simulink model "MdEnChk6s7s_Caller"  (R2018b)
settings: Solver=FixedStepDiscrete  StartTime=0.0  StopTime=10.0  RelTol=1e-3
undefined symbols (not defined in the file or in its folder): ChkBsyBit, MdAvl, MdEnChk6s7s_MdXX_Cal, Req, SetBsyBit, SetEnBit
libraries: simulink x6
settings Model: Creator=sn2xws  LastModifiedBy=sn2xws
settings DataIOCC: SaveFormat=StructureWithTime
settings OptimizationCC: DefaultParameterBehavior=Inlined  EnhancedBackFolding=on  PassReuseOutputArgsAs=Individual arguments  ZeroExternalMemoryAtStartup=off  ZeroInternalMemoryAtStartup=off  OptimizeBlockOrder=speed  DifferentSizesBufferReuse=on  OptimizationCustomize=off
settings DebuggingCC: ParameterTunabilityLossMsg=error
settings SFSimCC: MATLABDynamicMemAlloc=off
settings RTWCC: SystemTargetFile=autosar.tlc  GenCodeOnly=on  TemplateMakefile=ert_default_tmf  Description=AUTOSAR  GenerateReport=on  IncludeHyperlinkInReport=on  LaunchReport=on  GenerateTraceInfo=on  GenerateTraceReport=on  GenerateTraceReportSl=on  GenerateTraceReportSf=on  GenerateTraceReportEml=on  GenerateCodeMetricsReport=on
settings CodeAppCC: ForceParamTrailComments=on  IgnoreCustomStorageClasses=off  OperatorAnnotations=on  SimulinkDataObjDesc=on  SFDataObjDesc=on  InsertBlockDesc=on
settings STFCustomTargetCC: TargetLangStandard=C99 (ISO)  MultiwordLength=256  ParMdlRefBuildCompliant=on  CompOptLevelCompliant=on  IncludeMdlTerminateFcn=off  CombineOutputUpdateFcns=on  SuppressErrorStatus=on  ERTCustomFileBanners=on  SupportNonFinite=off  SupportComplex=off  SupportContinuousTime=off  SupportNonInlinedSFcns=off  RemoveResetFunc=on  MATLABClassNameForMDSCustomization=Simulink.SoftwareTarget.ERTCustomization  AutosarCompliant=on  UseToolchainInfoCompliant=on  LookupTableObjectStructAxisOrder=2,1,3,4,...  LUTObjectStructOrderEvenSpacing=Size,Table,Breakpoints  SystemTargetFile=autosar.tlc
settings ERTTargetCC: TargetLangStandard=C99 (ISO)  ConcurrentExecutionCompliant=off  IncludeMdlTerminateFcn=off  SuppressErrorStatus=on  SupportNonFinite=off  SupportComplex=off  ModelStepFunctionPrototypeControlCompliant=off  CPPClassGenCompliant=off  AutosarCompliant=on  LookupTableObjectStructAxisOrder=2,1,3,4,...  LUTObjectStructOrderEvenSpacing=Size,Table,Breakpoints  InlinedParameterPlacement=NonHierarchical  ERTCustomFileTemplate=example_file_process.tlc  ERTFilePackagingFormat=Compact

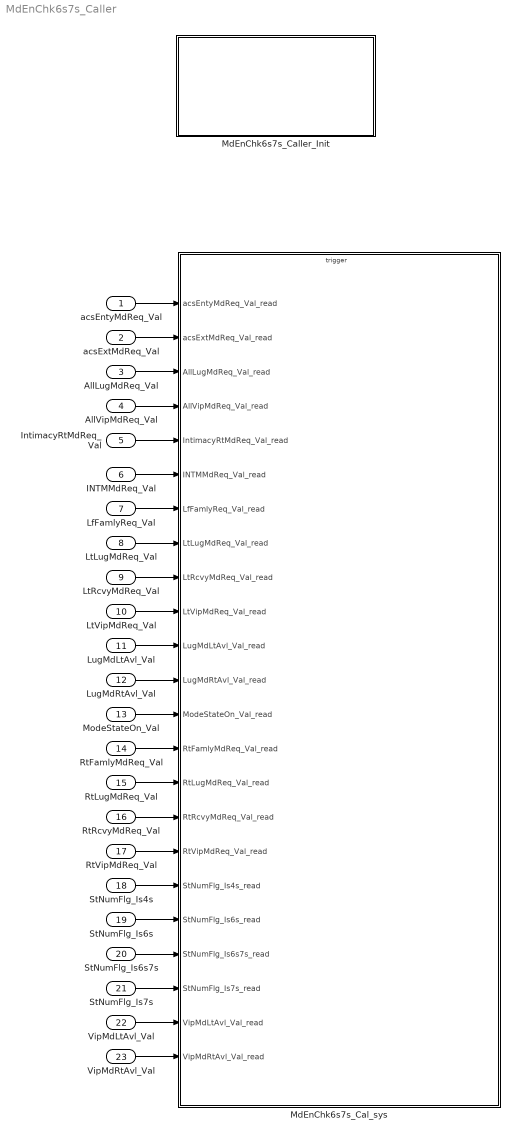
== system MdEnChk6s7s_Caller ==
  acsEntyMdReq_Val : Inport  OutDataTypeStr=boolean  PortDimensions=1
  acsExtMdReq_Val : Inport  Port=2  OutDataTypeStr=boolean  PortDimensions=1
  AllLugMdReq_Val : Inport  Port=3  OutDataTypeStr=boolean  PortDimensions=1
  AllVipMdReq_Val : Inport  Port=4  OutDataTypeStr=boolean  PortDimensions=1
  IntimacyRtMdReq_Val : Inport  Port=5  OutDataTypeStr=boolean  PortDimensions=1
  INTMMdReq_Val : Inport  Port=6  OutDataTypeStr=boolean  PortDimensions=1
  LfFamlyReq_Val : Inport  Port=7  OutDataTypeStr=boolean  PortDimensions=1
  LtLugMdReq_Val : Inport  Port=8  OutDataTypeStr=boolean  PortDimensions=1
  LtRcvyMdReq_Val : Inport  Port=9  OutDataTypeStr=boolean  PortDimensions=1
  LtVipMdReq_Val : Inport  Port=10  OutDataTypeStr=boolean  PortDimensions=1
  LugMdLtAvl_Val : Inport  Port=11  OutDataTypeStr=boolean  PortDimensions=1
  LugMdRtAvl_Val : Inport  Port=12  OutDataTypeStr=boolean  PortDimensions=1
  ModeStateOn_Val : Inport  Port=13  OutDataTypeStr=boolean  PortDimensions=1
  RtFamlyMdReq_Val : Inport  Port=14  OutDataTypeStr=boolean  PortDimensions=1
  RtLugMdReq_Val : Inport  Port=15  OutDataTypeStr=boolean  PortDimensions=1
  RtRcvyMdReq_Val : Inport  Port=16  OutDataTypeStr=boolean  PortDimensions=1
  RtVipMdReq_Val : Inport  Port=17  OutDataTypeStr=boolean  PortDimensions=1
  StNumFlg_Is4s : Inport  Port=18  OutDataTypeStr=boolean  PortDimensions=1
  StNumFlg_Is6s : Inport  Port=19  OutDataTypeStr=boolean  PortDimensions=1
  StNumFlg_Is6s7s : Inport  Port=20  OutDataTypeStr=boolean  PortDimensions=1
  StNumFlg_Is7s : Inport  Port=21  OutDataTypeStr=boolean  PortDimensions=1
  VipMdLtAvl_Val : Inport  Port=22  OutDataTypeStr=boolean  PortDimensions=1
  VipMdRtAvl_Val : Inport  Port=23  OutDataTypeStr=boolean  PortDimensions=1
  MdEnChk6s7s_Cal_sys : Subsystem
  MdEnChk6s7s_Caller_Init : Subsystem
  wires:
  acsEntyMdReq_Val/1 -> MdEnChk6s7s_Cal_sys/1(acsEntyMdReq_Val_read)
  acsExtMdReq_Val/1 -> MdEnChk6s7s_Cal_sys/2(acsExtMdReq_Val_read)
  AllLugMdReq_Val/1 -> MdEnChk6s7s_Cal_sys/3(AllLugMdReq_Val_read)
  AllVipMdReq_Val/1 -> MdEnChk6s7s_Cal_sys/4(AllVipMdReq_Val_read)
  IntimacyRtMdReq_Val/1 -> MdEnChk6s7s_Cal_sys/5(IntimacyRtMdReq_Val_read)
  INTMMdReq_Val/1 -> MdEnChk6s7s_Cal_sys/6(INTMMdReq_Val_read)
  LfFamlyReq_Val/1 -> MdEnChk6s7s_Cal_sys/7(LfFamlyReq_Val_read)
  LtLugMdReq_Val/1 -> MdEnChk6s7s_Cal_sys/8(LtLugMdReq_Val_read)
  LtRcvyMdReq_Val/1 -> MdEnChk6s7s_Cal_sys/9(LtRcvyMdReq_Val_read)
  LtVipMdReq_Val/1 -> MdEnChk6s7s_Cal_sys/10(LtVipMdReq_Val_read)
  LugMdLtAvl_Val/1 -> MdEnChk6s7s_Cal_sys/11(LugMdLtAvl_Val_read)
  LugMdRtAvl_Val/1 -> MdEnChk6s7s_Cal_sys/12(LugMdRtAvl_Val_read)
  ModeStateOn_Val/1 -> MdEnChk6s7s_Cal_sys/13(ModeStateOn_Val_read)
  RtFamlyMdReq_Val/1 -> MdEnChk6s7s_Cal_sys/14(RtFamlyMdReq_Val_read)
  RtLugMdReq_Val/1 -> MdEnChk6s7s_Cal_sys/15(RtLugMdReq_Val_read)
  RtRcvyMdReq_Val/1 -> MdEnChk6s7s_Cal_sys/16(RtRcvyMdReq_Val_read)
  RtVipMdReq_Val/1 -> MdEnChk6s7s_Cal_sys/17(RtVipMdReq_Val_read)
  StNumFlg_Is4s/1 -> MdEnChk6s7s_Cal_sys/18(StNumFlg_Is4s_read)
  StNumFlg_Is6s/1 -> MdEnChk6s7s_Cal_sys/19(StNumFlg_Is6s_read)
  StNumFlg_Is6s7s/1 -> MdEnChk6s7s_Cal_sys/20(StNumFlg_Is6s7s_read)
  StNumFlg_Is7s/1 -> MdEnChk6s7s_Cal_sys/21(StNumFlg_Is7s_read)
  VipMdLtAvl_Val/1 -> MdEnChk6s7s_Cal_sys/22(VipMdLtAvl_Val_read)
  VipMdRtAvl_Val/1 -> MdEnChk6s7s_Cal_sys/23(VipMdRtAvl_Val_read)

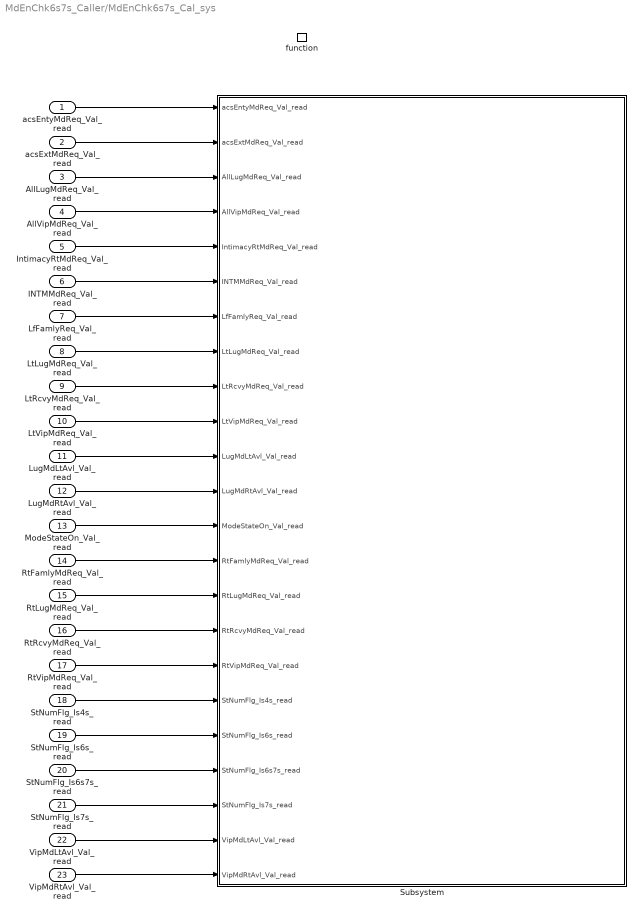
== system MdEnChk6s7s_Caller/MdEnChk6s7s_Cal_sys ==
  acsEntyMdReq_Val_read : Inport
  acsExtMdReq_Val_read : Inport  Port=2
  AllLugMdReq_Val_read : Inport  Port=3
  AllVipMdReq_Val_read : Inport  Port=4
  IntimacyRtMdReq_Val_read : Inport  Port=5
  INTMMdReq_Val_read : Inport  Port=6
  LfFamlyReq_Val_read : Inport  Port=7
  LtLugMdReq_Val_read : Inport  Port=8
  LtRcvyMdReq_Val_read : Inport  Port=9
  LtVipMdReq_Val_read : Inport  Port=10
  LugMdLtAvl_Val_read : Inport  Port=11
  LugMdRtAvl_Val_read : Inport  Port=12
  ModeStateOn_Val_read : Inport  Port=13
  RtFamlyMdReq_Val_read : Inport  Port=14
  RtLugMdReq_Val_read : Inport  Port=15
  RtRcvyMdReq_Val_read : Inport  Port=16
  RtVipMdReq_Val_read : Inport  Port=17
  StNumFlg_Is4s_read : Inport  Port=18
  StNumFlg_Is6s_read : Inport  Port=19
  StNumFlg_Is6s7s_read : Inport  Port=20
  StNumFlg_Is7s_read : Inport  Port=21
  VipMdLtAvl_Val_read : Inport  Port=22
  VipMdRtAvl_Val_read : Inport  Port=23
  function : TriggerPort  TriggerType=function-call  IsSimulinkFunction=on  FunctionName=MdEnChk6s7s_Cal  VariantControl=(inherit)
  Subsystem : Subsystem
  wires:
  acsEntyMdReq_Val_read/1 -> Subsystem/1(acsEntyMdReq_Val_read)
  acsExtMdReq_Val_read/1 -> Subsystem/2(acsExtMdReq_Val_read)
  AllLugMdReq_Val_read/1 -> Subsystem/3(AllLugMdReq_Val_read)
  AllVipMdReq_Val_read/1 -> Subsystem/4(AllVipMdReq_Val_read)
  IntimacyRtMdReq_Val_read/1 -> Subsystem/5(IntimacyRtMdReq_Val_read)
  INTMMdReq_Val_read/1 -> Subsystem/6(INTMMdReq_Val_read)
  LfFamlyReq_Val_read/1 -> Subsystem/7(LfFamlyReq_Val_read)
  LtLugMdReq_Val_read/1 -> Subsystem/8(LtLugMdReq_Val_read)
  LtRcvyMdReq_Val_read/1 -> Subsystem/9(LtRcvyMdReq_Val_read)
  LtVipMdReq_Val_read/1 -> Subsystem/10(LtVipMdReq_Val_read)
  LugMdLtAvl_Val_read/1 -> Subsystem/11(LugMdLtAvl_Val_read)
  LugMdRtAvl_Val_read/1 -> Subsystem/12(LugMdRtAvl_Val_read)
  ModeStateOn_Val_read/1 -> Subsystem/13(ModeStateOn_Val_read)
  RtFamlyMdReq_Val_read/1 -> Subsystem/14(RtFamlyMdReq_Val_read)
  RtLugMdReq_Val_read/1 -> Subsystem/15(RtLugMdReq_Val_read)
  RtRcvyMdReq_Val_read/1 -> Subsystem/16(RtRcvyMdReq_Val_read)
  RtVipMdReq_Val_read/1 -> Subsystem/17(RtVipMdReq_Val_read)
  StNumFlg_Is4s_read/1 -> Subsystem/18(StNumFlg_Is4s_read)
  StNumFlg_Is6s_read/1 -> Subsystem/19(StNumFlg_Is6s_read)
  StNumFlg_Is6s7s_read/1 -> Subsystem/20(StNumFlg_Is6s7s_read)
  StNumFlg_Is7s_read/1 -> Subsystem/21(StNumFlg_Is7s_read)
  VipMdLtAvl_Val_read/1 -> Subsystem/22(VipMdLtAvl_Val_read)
  VipMdRtAvl_Val_read/1 -> Subsystem/23(VipMdRtAvl_Val_read)

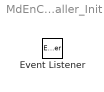
== system MdEnChk6s7s_Caller/MdEnChk6s7s_Caller_Init ==
  Event Listener : EventListener  EventName=reset

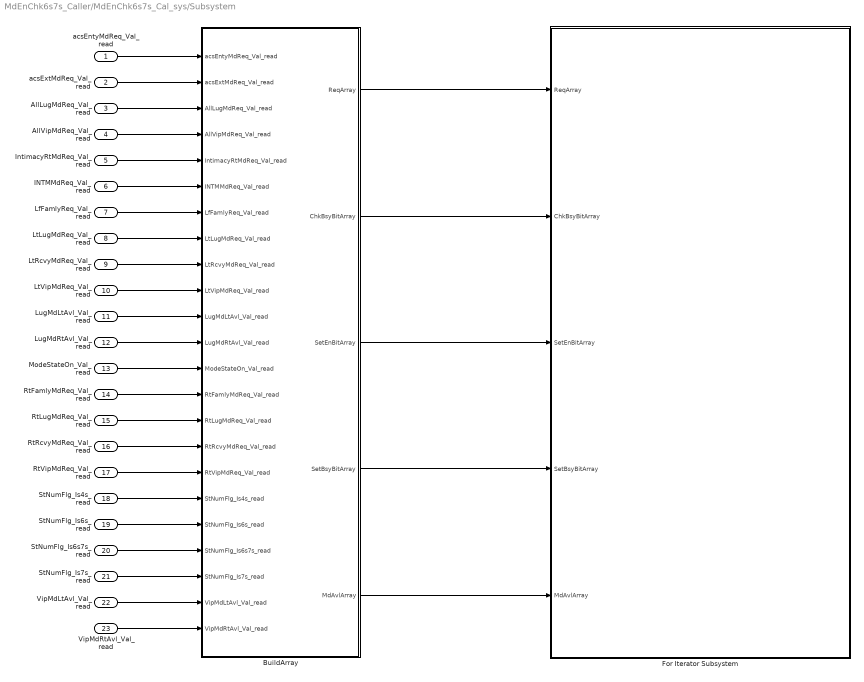
== system MdEnChk6s7s_Caller/MdEnChk6s7s_Cal_sys/Subsystem ==
  acsEntyMdReq_Val_read : Inport
  acsExtMdReq_Val_read : Inport  Port=2
  AllLugMdReq_Val_read : Inport  Port=3
  AllVipMdReq_Val_read : Inport  Port=4
  IntimacyRtMdReq_Val_read : Inport  Port=5
  INTMMdReq_Val_read : Inport  Port=6
  LfFamlyReq_Val_read : Inport  Port=7
  LtLugMdReq_Val_read : Inport  Port=8
  LtRcvyMdReq_Val_read : Inport  Port=9
  LtVipMdReq_Val_read : Inport  Port=10
  LugMdLtAvl_Val_read : Inport  Port=11
  LugMdRtAvl_Val_read : Inport  Port=12
  ModeStateOn_Val_read : Inport  Port=13
  RtFamlyMdReq_Val_read : Inport  Port=14
  RtLugMdReq_Val_read : Inport  Port=15
  RtRcvyMdReq_Val_read : Inport  Port=16
  RtVipMdReq_Val_read : Inport  Port=17
  StNumFlg_Is4s_read : Inport  Port=18
  StNumFlg_Is6s_read : Inport  Port=19
  StNumFlg_Is6s7s_read : Inport  Port=20
  StNumFlg_Is7s_read : Inport  Port=21
  VipMdLtAvl_Val_read : Inport  Port=22
  VipMdRtAvl_Val_read : Inport  Port=23
  BuildArray : Subsystem
  For Iterator Subsystem : Subsystem  TreatAsAtomicUnit=on
  wires:
  acsEntyMdReq_Val_read/1 -> BuildArray/1(acsEntyMdReq_Val_read)
  acsExtMdReq_Val_read/1 -> BuildArray/2(acsExtMdReq_Val_read)
  AllLugMdReq_Val_read/1 -> BuildArray/3(AllLugMdReq_Val_read)
  AllVipMdReq_Val_read/1 -> BuildArray/4(AllVipMdReq_Val_read)
  IntimacyRtMdReq_Val_read/1 -> BuildArray/5(IntimacyRtMdReq_Val_read)
  INTMMdReq_Val_read/1 -> BuildArray/6(INTMMdReq_Val_read)
  LfFamlyReq_Val_read/1 -> BuildArray/7(LfFamlyReq_Val_read)
  LtLugMdReq_Val_read/1 -> BuildArray/8(LtLugMdReq_Val_read)
  LtRcvyMdReq_Val_read/1 -> BuildArray/9(LtRcvyMdReq_Val_read)
  LtVipMdReq_Val_read/1 -> BuildArray/10(LtVipMdReq_Val_read)
  LugMdLtAvl_Val_read/1 -> BuildArray/11(LugMdLtAvl_Val_read)
  LugMdRtAvl_Val_read/1 -> BuildArray/12(LugMdRtAvl_Val_read)
  ModeStateOn_Val_read/1 -> BuildArray/13(ModeStateOn_Val_read)
  RtFamlyMdReq_Val_read/1 -> BuildArray/14(RtFamlyMdReq_Val_read)
  RtLugMdReq_Val_read/1 -> BuildArray/15(RtLugMdReq_Val_read)
  RtRcvyMdReq_Val_read/1 -> BuildArray/16(RtRcvyMdReq_Val_read)
  RtVipMdReq_Val_read/1 -> BuildArray/17(RtVipMdReq_Val_read)
  StNumFlg_Is4s_read/1 -> BuildArray/18(StNumFlg_Is4s_read)
  StNumFlg_Is6s_read/1 -> BuildArray/19(StNumFlg_Is6s_read)
  StNumFlg_Is6s7s_read/1 -> BuildArray/20(StNumFlg_Is6s7s_read)
  StNumFlg_Is7s_read/1 -> BuildArray/21(StNumFlg_Is7s_read)
  VipMdLtAvl_Val_read/1 -> BuildArray/22(VipMdLtAvl_Val_read)
  VipMdRtAvl_Val_read/1 -> BuildArray/23(VipMdRtAvl_Val_read)
  BuildArray/1(ReqArray) -> For Iterator Subsystem/1(ReqArray)
  BuildArray/2(ChkBsyBitArray) -> For Iterator Subsystem/2(ChkBsyBitArray)
  BuildArray/3(SetEnBitArray) -> For Iterator Subsystem/3(SetEnBitArray)
  BuildArray/4(SetBsyBitArray) -> For Iterator Subsystem/4(SetBsyBitArray)
  BuildArray/5(MdAvlArray) -> For Iterator Subsystem/5(MdAvlArray)

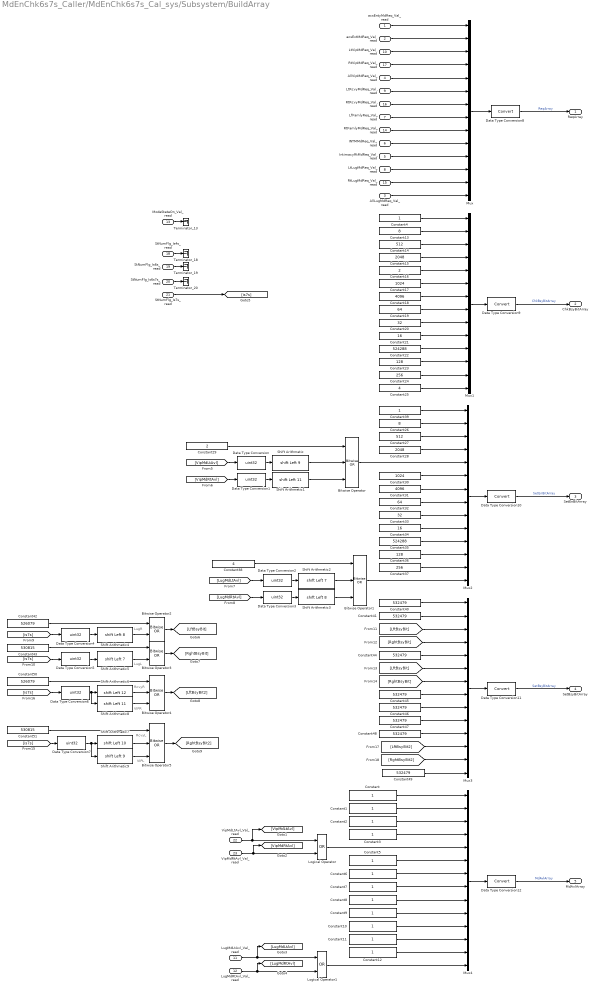
== system MdEnChk6s7s_Caller/MdEnChk6s7s_Cal_sys/Subsystem/BuildArray ==
  note: VIPR
  note: RcvyL
  note: VIPL
  note: RcvyR
  note: LugL
  note: LugR
  acsEntyMdReq_Val_read : Inport
  acsExtMdReq_Val_read : Inport  Port=2
  AllLugMdReq_Val_read : Inport  Port=3
  AllVipMdReq_Val_read : Inport  Port=4
  IntimacyRtMdReq_Val_read : Inport  Port=5
  INTMMdReq_Val_read : Inport  Port=6
  LfFamlyReq_Val_read : Inport  Port=7
  LtLugMdReq_Val_read : Inport  Port=8
  LtRcvyMdReq_Val_read : Inport  Port=9
  LtVipMdReq_Val_read : Inport  Port=10
  LugMdLtAvl_Val_read : Inport  Port=11
  LugMdRtAvl_Val_read : Inport  Port=12
  ModeStateOn_Val_read : Inport  Port=13
  RtFamlyMdReq_Val_read : Inport  Port=14
  RtLugMdReq_Val_read : Inport  Port=15
  RtRcvyMdReq_Val_read : Inport  Port=16
  RtVipMdReq_Val_read : Inport  Port=17
  StNumFlg_Is4s_read : Inport  Port=18
  StNumFlg_Is6s_read : Inport  Port=19
  StNumFlg_Is6s7s_read : Inport  Port=20
  StNumFlg_Is7s_read : Inport  Port=21
  VipMdLtAvl_Val_read : Inport  Port=22
  VipMdRtAvl_Val_read : Inport  Port=23
  Bitwise Operator{,1,4..5} (4 alike) : simulink/Logic and Bit Operations/Bitwise Operator  logicop=OR  UseBitMask=off  NumInputPorts=3  BitMask=bin2dec('11011001')  BitMaskRealWorld=Stored Integer
  Bitwise Operator2 : simulink/Logic and Bit Operations/Bitwise Operator  logicop=OR  UseBitMask=off  NumInputPorts=2  BitMask=bin2dec('11011001')  BitMaskRealWorld=Stored Integer
  Bitwise Operator3 : simulink/Logic and Bit Operations/Bitwise Operator  logicop=OR  UseBitMask=off  NumInputPorts=2  BitMask=bin2dec('11011001')  BitMaskRealWorld=Stored Integer
  Constant{,1..3,5..12} (12 alike) : Constant  OutDataTypeStr=boolean
  Constant13 : Constant  Value=8  OutDataTypeStr=uint32
  Constant14 : Constant  Value=512  OutDataTypeStr=uint32
  Constant15 : Constant  Value=2048  OutDataTypeStr=uint32
  Constant16 : Constant  Value=2  OutDataTypeStr=uint32
  Constant17 : Constant  Value=1024  OutDataTypeStr=uint32
  Constant18 : Constant  Value=4096  OutDataTypeStr=uint32
  Constant19 : Constant  Value=64  OutDataTypeStr=uint32
  Constant20 : Constant  Value=32  OutDataTypeStr=uint32
  Constant21 : Constant  Value=16  OutDataTypeStr=uint32
  Constant22 : Constant  Value=524288  OutDataTypeStr=uint32
  Constant23 : Constant  Value=128  OutDataTypeStr=uint32
  Constant24 : Constant  Value=256  OutDataTypeStr=uint32
  Constant25 : Constant  Value=4  OutDataTypeStr=uint32
  Constant26 : Constant  Value=8  OutDataTypeStr=uint32
  Constant27 : Constant  Value=512  OutDataTypeStr=uint32
  Constant28 : Constant  Value=2048  OutDataTypeStr=uint32
  Constant29 : Constant  Value=2  OutDataTypeStr=uint32
  Constant30 : Constant  Value=1024  OutDataTypeStr=uint32
  Constant31 : Constant  Value=4096  OutDataTypeStr=uint32
  Constant32 : Constant  Value=64  OutDataTypeStr=uint32
  Constant33 : Constant  Value=32  OutDataTypeStr=uint32
  Constant34 : Constant  Value=16  OutDataTypeStr=uint32
  Constant35 : Constant  Value=524288  OutDataTypeStr=uint32
  Constant36 : Constant  Value=128  OutDataTypeStr=uint32
  Constant37 : Constant  Value=256  OutDataTypeStr=uint32
  Constant38 : Constant  Value=4  OutDataTypeStr=uint32
  Constant39 : Constant  OutDataTypeStr=uint32
  Constant4 : Constant  OutDataTypeStr=uint32
  Constant{40..41,44..49} (8 alike) : Constant  Value=532479  OutDataTypeStr=uint32
  Constant42 : Constant  Value=526079  OutDataTypeStr=uint32
  Constant43 : Constant  Value=530815  OutDataTypeStr=uint32
  Constant50 : Constant  Value=526079  OutDataTypeStr=uint32
  Constant51 : Constant  Value=530815  OutDataTypeStr=uint32
  Data Type Conversion{,1..7} (8 alike) : DataTypeConversion  OutDataTypeStr=uint32
  Data Type Conversion{8..12} (5 alike) : DataTypeConversion
  Logical Operator : Logic  Operator=OR  AllPortsSameDT=off  OutDataTypeStr=boolean
  Logical Operator1 : Logic  Operator=OR  AllPortsSameDT=off  OutDataTypeStr=boolean
  Mux{,1..4} (5 alike) : Mux  Inputs=14
  Shift Arithmetic : ArithShift  BitShiftNumber=9  BitShiftDirection=Left
  Shift Arithmetic1 : ArithShift  BitShiftNumber=11  BitShiftDirection=Left
  Shift Arithmetic2 : ArithShift  BitShiftNumber=7  BitShiftDirection=Left
  Shift Arithmetic3 : ArithShift  BitShiftNumber=8  BitShiftDirection=Left
  Shift Arithmetic4 : ArithShift  BitShiftNumber=8  BitShiftDirection=Left
  Shift Arithmetic5 : ArithShift  BitShiftNumber=7  BitShiftDirection=Left
  Shift Arithmetic6 : ArithShift  BitShiftNumber=12  BitShiftDirection=Left
  Shift Arithmetic7 : ArithShift  BitShiftNumber=10  BitShiftDirection=Left
  Shift Arithmetic8 : ArithShift  BitShiftNumber=11  BitShiftDirection=Left
  Shift Arithmetic9 : ArithShift  BitShiftNumber=9  BitShiftDirection=Left
  Terminator_{13,18..20} (4 alike) : Terminator
  ReqArray : Outport
  ChkBsyBitArray : Outport  Port=2
  SetEnBitArray : Outport  Port=3
  SetBsyBitArray : Outport  Port=4
  MdAvlArray : Outport  Port=5
  wires:
  Constant43/1 -> Bitwise Operator3/1
  Shift Arithmetic5/1 -> Bitwise Operator3/2
  Constant42/1 -> Bitwise Operator2/1
  [LftBsyBit] -> Mux3/3
  Constant2/1 -> Mux4/3
  [RghtBsyBit2] -> Mux3/13
  Data Type Conversion3/1 -> Shift Arithmetic3/1
  Bitwise Operator2/1 -> [LftBsyBit]
  StNumFlg_Is7s_read/1 -> [is7s]
  Bitwise Operator5/1 -> [RghtBsyBit2]
  [LugMdRtAvl] -> Data Type Conversion3/1
  Constant12/1 -> Mux4/13
  [LugMdLtAvl] -> Data Type Conversion2/1
  Constant10/1 -> Mux4/11
  Constant8/1 -> Mux4/9
  Constant7/1 -> Mux4/8
  Constant6/1 -> Mux4/7
  Constant24/1 -> Mux1/13
  Constant25/1 -> Mux1/14
  Constant23/1 -> Mux1/12
  Constant22/1 -> Mux1/11
  Constant21/1 -> Mux1/10
  Constant20/1 -> Mux1/9
  Constant19/1 -> Mux1/8
  Constant18/1 -> Mux1/7
  Constant17/1 -> Mux1/6
  Constant15/1 -> Mux1/4
  Constant16/1 -> Mux1/5
  Constant14/1 -> Mux1/3
  [LftBsyBit2] -> Mux3/12
  IntimacyRtMdReq_Val_read/1 -> Mux/11
  acsExtMdReq_Val_read/1 -> Mux/2
  LfFamlyReq_Val_read/1 -> Mux/8
  Constant/1 -> Mux4/1
  Constant40/1 -> Mux3/1
  [RghtBsyBit] -> Mux3/4
  Shift Arithmetic6/1 -> Bitwise Operator4/2
  Mux3/1 -> Data Type Conversion11/1
  Constant49/1 -> Mux3/14
  Shift Arithmetic3/1 -> Bitwise Operator1/3
  Shift Arithmetic2/1 -> Bitwise Operator1/2
  Data Type Conversion5/1 -> Shift Arithmetic5/1
  VipMdLtAvl_Val_read/1 -> [VipMdLtAvl], Logical Operator/1
  Logical Operator/1 -> Mux4/5
  Logical Operator1/1 -> Mux4/14
  Bitwise Operator4/1 -> [LftBsyBit2]
  StNumFlg_Is6s_read/1 -> Terminator_19/1
  StNumFlg_Is4s_read/1 -> Terminator_18/1
  ModeStateOn_Val_read/1 -> Terminator_13/1
  Constant47/1 -> Mux3/10
  Constant1/1 -> Mux4/2
  StNumFlg_Is6s7s_read/1 -> Terminator_20/1
  Constant3/1 -> Mux4/4
  Data Type Conversion4/1 -> Shift Arithmetic4/1
  [LftBsyBit] -> Mux3/6
  RtRcvyMdReq_Val_read/1 -> Mux/7
  Mux2/1 -> Data Type Conversion10/1
  [RghtBsyBit] -> Mux3/7
  Constant38/1 -> Bitwise Operator1/1
  LtVipMdReq_Val_read/1 -> Mux/3
  RtVipMdReq_Val_read/1 -> Mux/4
  RtLugMdReq_Val_read/1 -> Mux/13
  LugMdLtAvl_Val_read/1 -> [LugMdLtAvl], Logical Operator1/1
  Constant29/1 -> Bitwise Operator/1
  Bitwise Operator/1 -> Mux2/5
  Shift Arithmetic1/1 -> Bitwise Operator/3
  Shift Arithmetic/1 -> Bitwise Operator/2
  [is7s] -> Data Type Conversion5/1
  AllLugMdReq_Val_read/1 -> Mux/14
  LtRcvyMdReq_Val_read/1 -> Mux/6
  Mux4/1 -> Data Type Conversion12/1
  LtLugMdReq_Val_read/1 -> Mux/12
  [is7s] -> Data Type Conversion6/1
  Bitwise Operator3/1 -> [RghtBsyBit]
  Bitwise Operator1/1 -> Mux2/14
  RtFamlyMdReq_Val_read/1 -> Mux/9
  Shift Arithmetic7/1 -> Bitwise Operator5/2
  Data Type Conversion7/1 -> Shift Arithmetic9/1, Shift Arithmetic7/1
  Shift Arithmetic9/1 -> Bitwise Operator5/3
  VipMdRtAvl_Val_read/1 -> Logical Operator/2, [VipMdRtAvl]
  Constant45/1 -> Mux3/8
  Constant9/1 -> Mux4/10
  Data Type Conversion2/1 -> Shift Arithmetic2/1
  Constant51/1 -> Bitwise Operator5/1
  Constant41/1 -> Mux3/2
  Constant11/1 -> Mux4/12
  acsEntyMdReq_Val_read/1 -> Mux/1
  [VipMdRtAvl] -> Data Type Conversion1/1
  Constant48/1 -> Mux3/11
  Constant46/1 -> Mux3/9
  Constant50/1 -> Bitwise Operator4/1
  Constant4/1 -> Mux1/1
  Shift Arithmetic8/1 -> Bitwise Operator4/3
  Data Type Conversion6/1 -> Shift Arithmetic8/1, Shift Arithmetic6/1
  Data Type Conversion/1 -> Shift Arithmetic/1
  AllVipMdReq_Val_read/1 -> Mux/5
  [is7s] -> Data Type Conversion4/1
  [VipMdLtAvl] -> Data Type Conversion/1
  Constant34/1 -> Mux2/10
  LugMdRtAvl_Val_read/1 -> [LugMdRtAvl], Logical Operator1/2
  Mux1/1 -> Data Type Conversion9/1
  Constant31/1 -> Mux2/7
  Constant35/1 -> Mux2/11
  Constant33/1 -> Mux2/9
  Constant27/1 -> Mux2/3
  Data Type Conversion1/1 -> Shift Arithmetic1/1
  Constant36/1 -> Mux2/12
  Constant32/1 -> Mux2/8
  Constant28/1 -> Mux2/4
  Constant37/1 -> Mux2/13
  Constant26/1 -> Mux2/2
  Constant5/1 -> Mux4/6
  Constant13/1 -> Mux1/2
  Constant39/1 -> Mux2/1
  INTMMdReq_Val_read/1 -> Mux/10
  Constant44/1 -> Mux3/5
  Constant30/1 -> Mux2/6
  Shift Arithmetic4/1 -> Bitwise Operator2/2
  [is7s] -> Data Type Conversion7/1
  Mux/1 -> Data Type Conversion8/1
  Data Type Conversion8/1 -> ReqArray/1  "ReqArray"
  Data Type Conversion9/1 -> ChkBsyBitArray/1  "ChkBsyBitArray"
  Data Type Conversion10/1 -> SetEnBitArray/1  "SetEnBitArray"
  Data Type Conversion11/1 -> SetBsyBitArray/1  "SetBsyBitArray"
  Data Type Conversion12/1 -> MdAvlArray/1  "MdAvlArray"

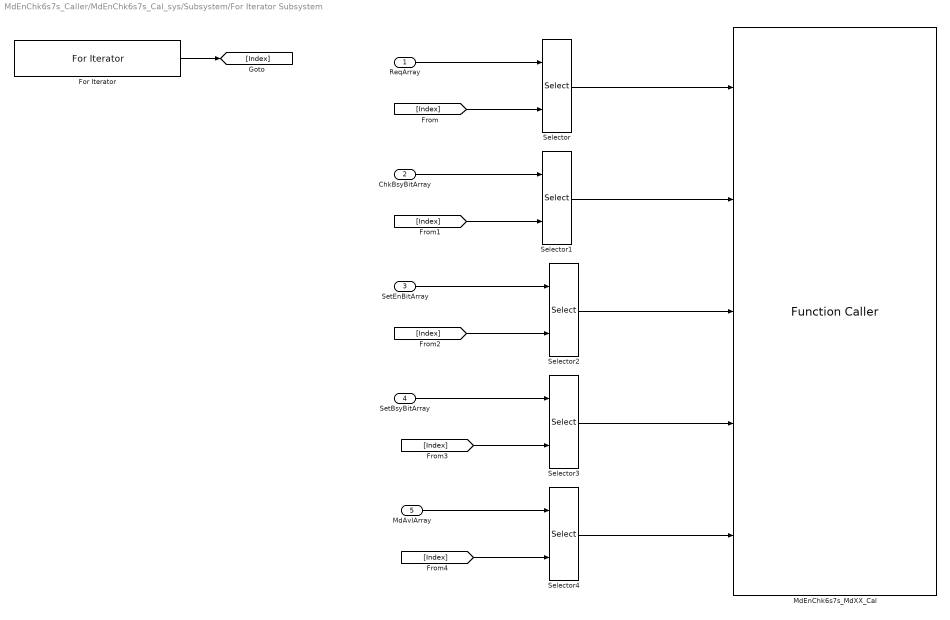
== system MdEnChk6s7s_Caller/MdEnChk6s7s_Cal_sys/Subsystem/For Iterator Subsystem ==
  ReqArray : Inport
  ChkBsyBitArray : Inport  Port=2
  SetEnBitArray : Inport  Port=3
  SetBsyBitArray : Inport  Port=4
  MdAvlArray : Inport  Port=5
  For Iterator : ForIterator  IterationLimit=14  IndexMode=Zero-based  IterationVariableDataType=int8
  MdEnChk6s7s_MdXX_Cal : FunctionCaller  Description=|  FunctionPrototype=MdEnChk6s7s_MdXX_Cal(Req,ChkBsyBit,SetEnBit,SetBsyBit,MdAvl)  InputArgumentSpecifications=boolean(true), uint32(1), uint32(1), uint32(1), boolean(true)
      | StNun: 
      | 0 :4s
      | 1:6s
      | 2:7s
      | 3:4sp
  Selector{,1..4} (5 alike) : Selector  IndexMode=Zero-based  InputPortWidth=14  IndexOptions=Index vector (port)  Indices=[1 3]  OutputSizes=1
  wires:
  For Iterator/1 -> [Index]
  [Index] -> Selector/2
  Selector/1 -> MdEnChk6s7s_MdXX_Cal/1
  [Index] -> Selector1/2
  Selector1/1 -> MdEnChk6s7s_MdXX_Cal/2
  Selector2/1 -> MdEnChk6s7s_MdXX_Cal/3
  [Index] -> Selector2/2
  [Index] -> Selector3/2
  [Index] -> Selector4/2
  Selector4/1 -> MdEnChk6s7s_MdXX_Cal/5
  Selector3/1 -> MdEnChk6s7s_MdXX_Cal/4
  ReqArray/1 -> Selector/1
  ChkBsyBitArray/1 -> Selector1/1
  SetEnBitArray/1 -> Selector2/1
  SetBsyBitArray/1 -> Selector3/1
  MdAvlArray/1 -> Selector4/1
